simulink model "BallAndBeamTS"  (R2018b)
settings: Solver=VariableStepAuto  StartTime=0.0  StopTime=ttotal  RelTol=1e-3
values from neighbouring files (symbols this model uses):
  alpha0 = -10*pi/180 + 20*pi/180 * rand    [IdentificacionTS.m]
  p0 = -0.25 + 0.5 * rand    [IdentificacionTS.m]
  tmuestra = 0.05    [ControlDeEstadosTS.m]    (also in IdentificacionTS.m; Otra_prueba_mas.m; Prueba.m)
  var = 0.001    [IdentificacionTS.m]    (also in Prueba.m = 1e-05)
undefined symbols (not defined in the file or in its folder): SimulBAB
settings Model: Creator=pablo  LastModifiedBy=pablo

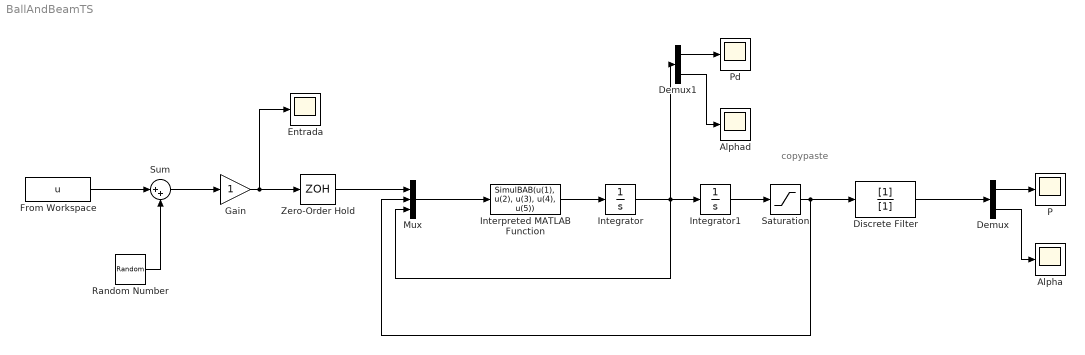
== system BallAndBeamTS ==
  note: copypaste
  "Alpha " : Scope
  Alphad : Scope
  Demux : Demux  Outputs=2
  Demux1 : Demux  Outputs=2
  Discrete Filter : DiscreteFilter  Denominator=[1]  SampleTime=tmuestra
  "Entrada " : Scope
  From Workspace : FromWorkspace  VariableName=u  SampleTime=tmuestra
  Gain : Gain
  Integrator : Integrator
  Integrator1 : Integrator  InitialCondition=[p0, alpha0]
  Interpreted MATLAB Function : MATLABFcn  MATLABFcn=SimulBAB(u(1), u(2), u(3), u(4), u(5))  OutputDimensions=2
  Mux : Mux  Inputs=3
  P : Scope
  Pd : Scope
  Random Number : RandomNumber  Variance=var  Seed=354872  SampleTime=tmuestra
  Saturation : Saturate  UpperLimit=[0.4; 15*pi/180]  LowerLimit=-[0.4; 15*pi/180]
  Sum : Sum  Inputs=|++
  Zero-Order Hold : ZeroOrderHold  SampleTime=tmuestra
  wires:
  From Workspace/1 -> Sum/1
  Random Number/1 -> Sum/2
  Gain/1 -> Zero-Order Hold/1, "Entrada "/1
  Sum/1 -> Gain/1
  Mux/1 -> Interpreted MATLAB Function/1
  Zero-Order Hold/1 -> Mux/1
  Interpreted MATLAB Function/1 -> Integrator/1
  Demux/2 -> "Alpha "/1
  Demux/1 -> P/1
  Integrator1/1 -> Saturation/1
  Saturation/1 -> Mux/2, Discrete Filter/1
  Discrete Filter/1 -> Demux/1
  Demux1/1 -> Pd/1
  Integrator/1 -> Demux1/1, Mux/3, Integrator1/1
  Demux1/2 -> Alphad/1
